simulink model "FFT_4096_length"  (R2020a)
settings: Solver=VariableStepAuto  StartTime=0.0  StopTime=((3*4096)-1)/1000  RelTol=1e-3
PreLoadFcn:
  | setenv("DSPLIB_ROOT",xmcLibraryPath('get','dsplib'))
undefined symbols (not defined in the file): aie, api_cast, dsp, S, vsva2197, widget, widget_api_cast_graph, xcvc1902, xf
libraries: ModelComposer x5, simulink x1, dspsrcs4 x1
settings Model: Creator=ravidapu  LastModifiedBy=viswanad

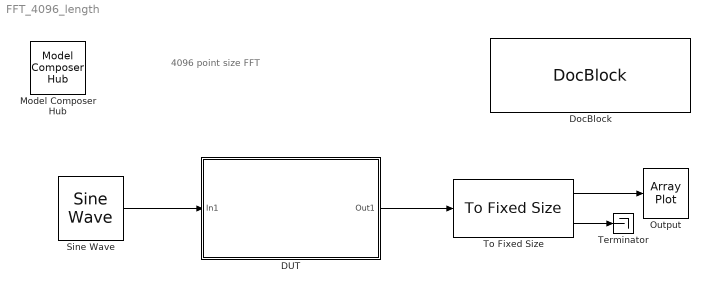
== system FFT_4096_length ==
  note: 4096 point size FFT
  DUT : Subsystem
  DocBlock : simulink/Model-Wide Utilities/DocBlock  DocumentType=Text  mask(DocBlock){}
      content=|
      | ///////////////////////////////////////////////////////////////////////////
      | // Copyright 2021 Xilinx
      | //
      | // Licensed under the Apache License, Version 2.0 (the "License");
      | // you may not use this file except in compliance with the License.
      | // You may obtain a copy of the License at
      | //
      | // http://www.apache.org/licenses/LICENSE-2.0
      | //
      | // Unless required by applicable law or agreed to in writing, software
      | // distributed under the License is distributed on an "AS IS" BASIS,
      | // WITHOUT WARRANTIES OR CONDITIONS OF ANY KIND, either express or implied.
      | // See the License for the specific language governing permissions and
      | // limitations under the License.
      | ///////////////////////////////////////////////////////////////////////////
      mask Display:
      | xmcDrawBlockIcon();
      | disp(['{\fontsize{10pt}(c) Copyright 2021' ' Xilinx, Inc.}\newline \newline '],'texmode','on');
      | disp('{\fontsize{10pt}Licensed under the Apache License 2.0}','texmode','on');
      | disp('\newline \newline \newline{\fontsize{10pt}Double Click for Copyright Notice}','texmode','on');
  Model Composer Hub : ModelComposer/Model Composer Hub  CodeGeneration=off  SubsystemName=DUT  TargetDirectory=./code  ExportType=AI Engines  IpVendor=xilinx.com  IpLibrary=hls  IpVersion=1.0  IpHWLanguage=Verilog  AieCompilerOptions={'-heapsize=8000'}  CreateTestbench=on  TestbenchStackSize=10  RunAieSim=on  AieSimTimeout=50000  RunAieSimProfiling=off  LaunchVitisAnalyzer=on  PlotOutput=off  RunX86Sim=off  X86SimTimeout=10  GenHwImage=off  PlatformType=Not Specified  ProjDevice=xcvc1902-vsva2197-2MP-e-S  ProjDevicePart=xcvc1902-vsva2197-2MP-e-S  SamplePeriod=-1  ClockFrequency=200  DataPathParallelism=1
  Output : ArrayPlot
  Sine Wave : dspsrcs4/Sine Wave  Amplitude=64  Frequency=200  Phase=0  SampleMode=Discrete  OutComplex=Complex  CompMethod=Table lookup  TableSize=Speed  SampleTime=1/1000  SamplesPerFrame=1  ResetState=Restart at time zero  OutputFrames=off  dataType=Fixed-point  wordLen=16  udDataType=sfix(16)  fracBitsMode=User-defined  numFracBits=0  OutDataTypeStr=fixdt(1,16,0)  LastOutDataTypeStr=fixdt(1,16,0)
  Terminator : Terminator
  To Fixed Size : ModelComposer/To Fixed Size  OutputSize=4096  CopyMethod=Buffer samples to form output  HasStatusOutput=off
  wires:
  Sine Wave/1 -> DUT/1(In1)
  To Fixed Size/1 -> Output/1
  To Fixed Size/2 -> Terminator/1
  DUT/1(Out1) -> To Fixed Size/1

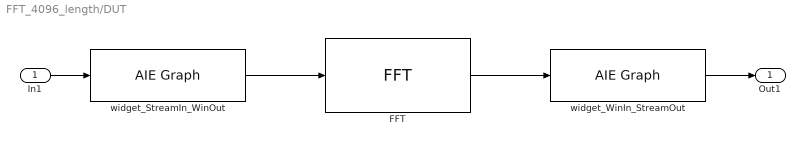
== system FFT_4096_length/DUT ==
  In1 : Inport
  FFT : ModelComposer/FFT  data_type=cint16  point_size=4096  input_window_size=4096  shift_val=0  input_sampling_rate=200  use_casc_length=on  casc_length=1  spec=meta_data_hl_fft.json
  widget_StreamIn_WinOut : ModelComposer/AIE Graph  PortAttributesTable={'Input', 'in[0]', 'stream', 'cint16', '', '', '';'Output', 'out[0]', 'window', 'cint16', '4096', 'sync', ''}  PortAttributesEnablement={'off', 'on', 'off', 'off', 'off', 'off', 'off';'off', 'on', 'off', 'off', 'off', 'off', 'off'}  SampleTime=-1  ClassDeclTypeOptions=C[1 1]@t224@template < typename TT_DATA, unsigned int TP_IN_API, unsigned int TP_OUT_API, unsigned int TP_NUM_INPUTS, unsigned int TP_WINDOW_VSIZE, unsigned int TP_NUM_OUTPUT_CLONES, unsigned int TP_PATTERN > class widget_api_cast_graph  ClassDecl=template < typename TT_DATA, unsigned int TP_IN_API, unsigned int TP_OUT_API, unsigned int TP_NUM_INPUTS, unsigned int TP_WINDOW_VSIZE, unsigned int TP_NUM_OUTPUT_CLONES, unsigned int TP_PATTERN > class widget_api_cast_graph  ClassTemplateParams={'TT_DATA', 'typename', 'cint16';'TP_IN_API', 'unsigned int', '1';'TP_OUT_API', 'unsigned int', '0';'TP_NUM_INPUTS', 'unsigned int', '1';'TP_WINDOW_VSIZE', 'unsigned int', '4096';'TP_NUM_OUTPUT_CLONES', 'unsigned int', '1';'TP_PATTERN', 'unsigned int', '0'}  ClassTemplateParamsEnables={'off', 'off', 'on';'off', 'off', 'on';'off', 'off', 'on';'off', 'off', 'on';'off', 'off', 'on';'off', 'off', 'on';'off', 'off', 'on'}  ClassPortParams={ 'input', 'in[TP_NUM_INPUTS]', 'off'; 'output', 'out[TP_NUM_OUTPUT_CLONES]', 'off' }  ClassCtorDeclTypeOptions=C[1 1]@t7@<empty>  ClassCtorDecl=<empty>  ClassCtorParams={}  GraphAllAttrs=|  PortArgDecls={'in stream cint16 in1'; 'out window cint16 out1'}  PortGraphPortNames={'in[0]'; 'out[0]'}  PortTypes={'stream'; 'window'}  PortDataTypes={'cint16'; 'cint16'}  PortSizes={0.000000000000000000e+00; 4.096000000000000000e+03}  PortSynchronicities={'auto'; 'sync'}  PortSignalSizes={0.000000000000000000e+00; 0.000000000000000000e+00}  SimLibPath=''  ClassIndex=1  ClassCtorIndex=0  ClassTabVisible=on  FunctionTabVisible=on  DelayDrawLabels=off  GraphFileSelect=Header file (*.h)  GraphHeaderFile=$DSPLIB_ROOT/L2/include/aie/widget_api_cast_graph.hpp  GraphClassName=xf::dsp::aie::widget::api_cast::widget_api_cast_graph  GraphName=xf::dsp::aie::widget::api_cast::widget_api_cast_graph<cint16, 1, 0, 1, 4096, 1, 0>  GraphHeaderFiles={'/proj/xbuilds/SWIP/2021.2_1006_2051/installs/lin64/Model_Composer/2021.2/tps/xf_dsp/L2/include/aie/widget_api_cast_graph.hpp'}  GraphSourceFile=./model_composer_work/xmc_aie_lib/a367e87c/mygraph.cpp  GraphSearchPaths={'$DSPLIB_ROOT/L2/include/aie', '$DSPLIB_ROOT/L1/include/aie/', '$DSPLIB_ROOT/L1/src/aie'}  GraphPreProcOptions={}  blockJsonConstraints=[]  deprecateConstraints=0
      | s[12;12;9;9;19;14;21;23;24;21;12;24;26;26;26;27;28;9;21;23;23;23;24;25;14;19;19;29]@FunctionNameDeclFileNamePortNamesPortTypesPortSerializedTypesPortDirectionsPortWindowSizeEnablesPortWindowMarginEnablesPortSynchronicityEnablesPortSignalSizeEnablesFunctionDeclFunctionTemplateSpecKindFunctionTemplateParamNamesFunctionTemplateParamKindsFunctionTemplateParamTypesFunctionTemplateParamValuesFunctionTemplateParamEnablesClassDeclClassTemplateSpecKindClassTemplateParamNamesClassTemplateParamKindsClassTemplateParamTypesClassTemplateParamValuesClassTemplateParamEnablesClassCtorDeclsClassCtorParamNamesClassCtorParamTypesClassCtorParamSerializedTypes[1 1]@C[28 1]@nt124@/proj/xbuilds/SWIP/2021.2_1006_2051/installs/lin64/Model_Composer/2021.2/tps/xf_dsp/L2/include/aie/widget_api_cast_graph.hppC[2 1]@t2@int3@outC[2 1]@t48@adf::port< adf::direction::in >[ TP_NUM_INPUTS ]t56@adf::port< adf::direction::out >[ TP_NUM_OUTPUT_CLONES ]C[2 1]@t55@{D{Tadf::port{1{t{Sadf::direction::in}}}}TP_NUM_INPUTS}t63@{D{Tadf::port{1{t{Sadf::direction::out}}}}TP_NUM_OUTPUT_CLONES}C[2 1]@t5@inputt5@inputC[2 1]@l0@l0@C[2 1]@l0@l0@C[2 1]@l1@l1@C[2 1]@l0@l0@t442@namespace xf { namespace dsp { namespace aie { namespace widget { namespace api_cast {
      | template < typename TT_DATA, unsigned int TP_IN_API, unsigned int TP_OUT_API, unsigned int TP_NUM_INPUTS, unsigned int TP_WINDOW_VSIZE, unsigned int TP_NUM_OUTPUT_CLONES, unsigned int TP_PATTERN > 
      | void widget_api_cast_graph::
      | (adf::port< adf::direction::in > in [ TP_NUM_INPUTS ], adf::port< adf::direction::out > out [ TP_NUM_OUTPUT_CLONES ]);
      | } } } } }ne[0 1]@e[0 1]@e[0 1]@e[0 1]@e[0 1]@t322@namespace xf { namespace dsp { namespace aie { namespace widget { namespace api_cast {
      | template < typename TT_DATA, unsigned int TP_IN_API, unsigned int TP_OUT_API, unsigned int TP_NUM_INPUTS, unsigned int TP_WINDOW_VSIZE, unsigned int TP_NUM_OUTPUT_CLONES, unsigned int TP_PATTERN > class widget_api_cast_graph;
      | } } } } }t8@implicitC[7 1]@t7@TT_DATAt9@TP_IN_APIt10@TP_OUT_APIt13@TP_NUM_INPUTSt15@TP_WINDOW_VSIZEt20@TP_NUM_OUTPUT_CLONESt10@TP_PATTERNC[7 1]@t4@typet7@nontypet7@nontypet7@nontypet7@nontypet7@nontypet7@nontypeC[7 1]@t8@typenamet12@unsigned intt12@unsigned intt12@unsigned intt12@unsigned intt12@unsigned intt12@unsigned intC[7 1]@nnnnnnnC[7 1]@l1@l1@l1@l1@l1@l1@l1@e[0 1]@e[0 1]@e[0 1]@e[0 1]@
  widget_WinIn_StreamOut : ModelComposer/AIE Graph  PortAttributesTable={ 'Input', 'in[0]', 'window', 'cint16', '4096', 'sync', ''; 'Output', 'out[0]', 'stream', 'cint16', '', '', '4096' }  PortAttributesEnablement={'off', 'on', 'off', 'off', 'off', 'off', 'off';'off', 'on', 'off', 'off', 'off', 'off', 'on'}  SampleTime=-1  ClassDeclTypeOptions=C[1 1]@t224@template < typename TT_DATA, unsigned int TP_IN_API, unsigned int TP_OUT_API, unsigned int TP_NUM_INPUTS, unsigned int TP_WINDOW_VSIZE, unsigned int TP_NUM_OUTPUT_CLONES, unsigned int TP_PATTERN > class widget_api_cast_graph  ClassDecl=template < typename TT_DATA, unsigned int TP_IN_API, unsigned int TP_OUT_API, unsigned int TP_NUM_INPUTS, unsigned int TP_WINDOW_VSIZE, unsigned int TP_NUM_OUTPUT_CLONES, unsigned int TP_PATTERN > class widget_api_cast_graph  ClassTemplateParams={'TT_DATA', 'typename', 'cint16';'TP_IN_API', 'unsigned int', '0';'TP_OUT_API', 'unsigned int', '1';'TP_NUM_INPUTS', 'unsigned int', '1';'TP_WINDOW_VSIZE', 'unsigned int', '4096';'TP_NUM_OUTPUT_CLONES', 'unsigned int', '1';'TP_PATTERN', 'unsigned int', '0'}  ClassTemplateParamsEnables={'off', 'off', 'on';'off', 'off', 'on';'off', 'off', 'on';'off', 'off', 'on';'off', 'off', 'on';'off', 'off', 'on';'off', 'off', 'on'}  ClassPortParams={ 'input', 'in[TP_NUM_INPUTS]', 'off'; 'output', 'out[TP_NUM_OUTPUT_CLONES]', 'off' }  ClassCtorDeclTypeOptions=C[1 1]@t7@<empty>  ClassCtorDecl=<empty>  ClassCtorParams={}  GraphAllAttrs=|  PortArgDecls={'in window cint16 in1'; 'out stream cint16 out1'}  PortGraphPortNames={'in[0]'; 'out[0]'}  PortTypes={'window'; 'stream'}  PortDataTypes={'cint16'; 'cint16'}  PortSizes={4.096000000000000000e+03; 0.000000000000000000e+00}  PortSynchronicities={'sync'; 'auto'}  PortSignalSizes={0.000000000000000000e+00; 4.096000000000000000e+03}  SimLibPath=''  ClassIndex=1  ClassCtorIndex=0  ClassTabVisible=on  FunctionTabVisible=on  DelayDrawLabels=off  GraphFileSelect=Header file (*.h)  GraphHeaderFile=$DSPLIB_ROOT/L2/include/aie/widget_api_cast_graph.hpp  GraphClassName=xf::dsp::aie::widget::api_cast::widget_api_cast_graph  GraphName=xf::dsp::aie::widget::api_cast::widget_api_cast_graph<cint16, 0, 1, 1, 4096, 1, 0>  GraphHeaderFiles={'/proj/xbuilds/SWIP/2021.2_1021_0703/installs/lin64/Model_Composer/2021.2/tps/xf_dsp/L2/include/aie/widget_api_cast_graph.hpp'}  GraphSourceFile=./model_composer_work/xmc_aie_lib/6a2360af/mygraph.cpp  GraphSearchPaths={'$DSPLIB_ROOT/L2/include/aie', '$DSPLIB_ROOT/L1/include/aie/', '$DSPLIB_ROOT/L1/src/aie'}  GraphPreProcOptions={}  blockJsonConstraints=[]  deprecateConstraints=0
      | s[12;12;9;9;19;14;21;23;24;21;12;24;26;26;26;27;28;9;21;23;23;23;24;25;14;19;19;29]@FunctionNameDeclFileNamePortNamesPortTypesPortSerializedTypesPortDirectionsPortWindowSizeEnablesPortWindowMarginEnablesPortSynchronicityEnablesPortSignalSizeEnablesFunctionDeclFunctionTemplateSpecKindFunctionTemplateParamNamesFunctionTemplateParamKindsFunctionTemplateParamTypesFunctionTemplateParamValuesFunctionTemplateParamEnablesClassDeclClassTemplateSpecKindClassTemplateParamNamesClassTemplateParamKindsClassTemplateParamTypesClassTemplateParamValuesClassTemplateParamEnablesClassCtorDeclsClassCtorParamNamesClassCtorParamTypesClassCtorParamSerializedTypes[1 1]@C[28 1]@nt124@/proj/xbuilds/SWIP/2021.2_1006_2051/installs/lin64/Model_Composer/2021.2/tps/xf_dsp/L2/include/aie/widget_api_cast_graph.hppC[2 1]@t2@int3@outC[2 1]@t48@adf::port< adf::direction::in >[ TP_NUM_INPUTS ]t56@adf::port< adf::direction::out >[ TP_NUM_OUTPUT_CLONES ]C[2 1]@t55@{D{Tadf::port{1{t{Sadf::direction::in}}}}TP_NUM_INPUTS}t63@{D{Tadf::port{1{t{Sadf::direction::out}}}}TP_NUM_OUTPUT_CLONES}C[2 1]@t5@inputt5@inputC[2 1]@l0@l0@C[2 1]@l0@l0@C[2 1]@l1@l1@C[2 1]@l0@l0@t442@namespace xf { namespace dsp { namespace aie { namespace widget { namespace api_cast {
      | template < typename TT_DATA, unsigned int TP_IN_API, unsigned int TP_OUT_API, unsigned int TP_NUM_INPUTS, unsigned int TP_WINDOW_VSIZE, unsigned int TP_NUM_OUTPUT_CLONES, unsigned int TP_PATTERN > 
      | void widget_api_cast_graph::
      | (adf::port< adf::direction::in > in [ TP_NUM_INPUTS ], adf::port< adf::direction::out > out [ TP_NUM_OUTPUT_CLONES ]);
      | } } } } }ne[0 1]@e[0 1]@e[0 1]@e[0 1]@e[0 1]@t322@namespace xf { namespace dsp { namespace aie { namespace widget { namespace api_cast {
      | template < typename TT_DATA, unsigned int TP_IN_API, unsigned int TP_OUT_API, unsigned int TP_NUM_INPUTS, unsigned int TP_WINDOW_VSIZE, unsigned int TP_NUM_OUTPUT_CLONES, unsigned int TP_PATTERN > class widget_api_cast_graph;
      | } } } } }t8@implicitC[7 1]@t7@TT_DATAt9@TP_IN_APIt10@TP_OUT_APIt13@TP_NUM_INPUTSt15@TP_WINDOW_VSIZEt20@TP_NUM_OUTPUT_CLONESt10@TP_PATTERNC[7 1]@t4@typet7@nontypet7@nontypet7@nontypet7@nontypet7@nontypet7@nontypeC[7 1]@t8@typenamet12@unsigned intt12@unsigned intt12@unsigned intt12@unsigned intt12@unsigned intt12@unsigned intC[7 1]@nnnnnnnC[7 1]@l1@l1@l1@l1@l1@l1@l1@e[0 1]@e[0 1]@e[0 1]@e[0 1]@
  Out1 : Outport
  wires:
  widget_StreamIn_WinOut/1 -> FFT/1
  In1/1 -> widget_StreamIn_WinOut/1
  FFT/1 -> widget_WinIn_StreamOut/1
  widget_WinIn_StreamOut/1 -> Out1/1
